simulink model "interval_step_function"  (R2019a)
settings: Solver=VariableStepAuto  StartTime=0.0  StopTime=10.0  RelTol=1e-3
settings Model: Creator=a3bawa  LastModifiedBy=a3bawa

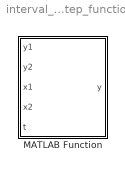
== system interval_step_function ==
  MATLAB Function : MATLAB Function  TreatAsAtomicUnit=on

== matlab function interval_step_function/MATLAB Function ==
  data: y1 input; y output; y2 input; x1 input; x2 input; t input
function y = fcn(y1,y2,x1,x2,t)

if (x1<=t)&&(t<x2)
    y=y1;
else
    y=y2;
end
